simulink model "C1f_sim"  (R2021b)
settings: Solver=VariableStepAuto  StartTime=0.0  StopTime=20  RelTol=1e-3
settings Model: Creator=Studenci  LastModifiedBy=Studenci

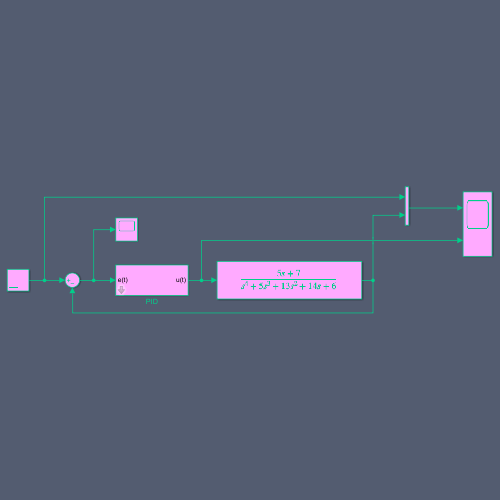
[thumbnail: Simulink's stored preview of the top-level diagram]
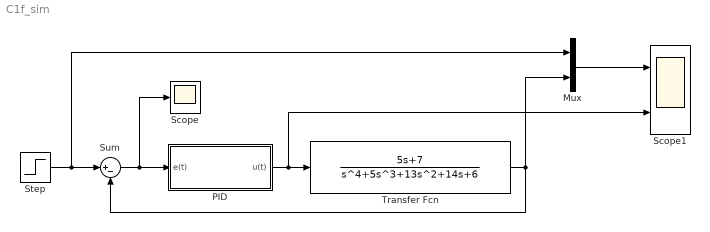
== system C1f_sim ==
  Mux : Mux  Inputs=2
  PID : Subsystem  mask{Kp=2.972367437761131, Ki=2.634595834216244, Kd=0.838360866429722}
      mask prompts: Kp "Kp ="; Ki "Ki ="; Kd "Kd ="
  Scope : Scope
  Scope1 : Scope  NumInputPorts=2
  Step : Step  Time=0  SampleTime=0.1
  Sum : Sum  Inputs=|+-
  Transfer Fcn : TransferFcn  Numerator=[5 7]  Denominator=[1 5 13 14 6]
  wires:
  Step/1 -> Mux/1, Sum/1
  Sum/1 -> PID/1(e(t)), Scope/1
  PID/1(u(t)) -> Transfer Fcn/1, Scope1/2
  Mux/1 -> Scope1/1
  Transfer Fcn/1 -> Mux/2, Sum/2

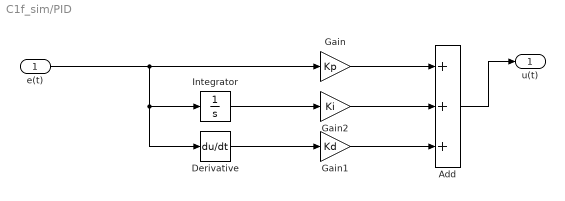
== system C1f_sim/PID ==
  e(t) : Inport
  Add : Sum  Inputs=+++
  Derivative : Derivative
  Gain : Gain  Gain=Kp
  Gain1 : Gain  Gain=Kd
  Gain2 : Gain  Gain=Ki
  Integrator : Integrator
  u(t) : Outport
  wires:
  e(t)/1 -> Derivative/1, Integrator/1, Gain/1
  Integrator/1 -> Gain2/1
  Derivative/1 -> Gain1/1
  Gain/1 -> Add/1
  Add/1 -> u(t)/1
  Gain2/1 -> Add/2
  Gain1/1 -> Add/3
